simulink model "fin_simu_continuous"  (R2022a)
settings: Solver=ode45  StartTime=0.0  StopTime=time  RelTol=1e-8  AbsTol=1e-10
values from neighbouring files (symbols this model uses):
  A0 = [0, 1; -1, -1.4]    [code_simu_continuous_simplified.m]    (also in matlab.mat = [0  1; -1  -1.4])
  AA_s = [-2.2  -10.2  -9; 1  0  0; 0  1  0]    [matlab.mat]
  AT = [0,1;-9,-1.2]    [code_simu.m]    (also in code_simu_continuous_simplified.m = [0, 1; -9, -1.2]; matlab.mat = [0  1; -9  -1.2])
  b0 = readmatrix('result_NNFF&ROB\20251002_153045\z2_biases_layer_0.csv','Range','A1:A30')    [getNN_simu.m]    (also in matlab.mat = [0.168317809701 -0.0711987838149 -0.0412988699973 -0.0729310)
  B0 = [0; 1]    [code_simu_continuous_simplified.m]    (also in matlab.mat = [0 1])
  b1 = readmatrix('result_NNFF&ROB\20251002_153045\z2_biases_layer_1.csv','Range','A1:A20')    [getNN_simu.m]    (also in matlab.mat = [-0.0446465238929 0.0289220847189 -0.0468313358724 -0.028365)
  b2 = readmatrix('result_NNFF&ROB\20251002_153045\z2_biases_layer_2.csv','Range','A1:A10')    [getNN_simu.m]    (also in matlab.mat = [-0.0184617917985 -0.0854043364525 -0.0408402681351 0.561344)
  b3 = readmatrix('result_NNFF&ROB\20251002_153045\z2_biases_layer_3.csv','Range','A1:A1')    [getNN_simu.m]    (also in matlab.mat = 0.3782748878)
  BB_s = [1 0 0]    [matlab.mat]
  BT = [0;1]    [code_simu.m]    (also in code_simu_continuous_simplified.m = [0; 1]; matlab.mat = [0 1])
  C0 = [1, 0]    [code_simu_continuous_simplified.m]    (also in matlab.mat = [1 0])
  CC_s = [-8.1 -30.42 -14.4]    [matlab.mat]
  CT = [22.5,9]    [code_simu.m]    (also in code_simu_continuous_simplified.m = [22.5, 9]; matlab.mat = [22.5 9])
  D0 = [0]    [code_simu_continuous_simplified.m]    (also in matlab.mat = 0)
  DD_s = 0.1    [matlab.mat]
  DT = 0    [code_simu.m]    (also in code_simu_continuous_simplified.m; matlab.mat)
  gamma = 2    [code_simu.m]    (also in code_simu_continuous_simplified.m = 1000; matlab.mat = 1000)
  omega = 3.14159265*5    (= 15.70796325)    [code_simu.m]    (also in code_simu_continuous_simplified.m; matlab.mat)
  ran_max = 20    [code_simu.m]    (also in code_simu_continuous_simplified.m; matlab.mat)
  ran_min = 5    [code_simu.m]    (also in code_simu_continuous_simplified.m; matlab.mat)
  rho = 0.101    [code_simu.m]    (also in code_simu_continuous_simplified.m = 0.3; matlab.mat = 0.5)
  seed = 17    [code_simu.m]    (also in code_simu_continuous_simplified.m = randi(2^31-2); matlab.mat = 2084332126)
  sigma = 10    [code_simu.m]    (also in code_simu_continuous_simplified.m = 0.1; matlab.mat = 100)
  Td = 0.001    [code_simu_continuous_simplified.m]    (also in matlab.mat)
  w0 = readmatrix('result_NNFF&ROB\20251002_153045\z2_weights_layer_0.csv','Range','A1:AD4')    [getNN_simu.m]    (also in matlab.mat = [0.408856898546 -0.0425847135484 0.404223948717 0.4036423563)
  w1 = readmatrix('result_NNFF&ROB\20251002_153045\z2_weights_layer_1.csv','Range','A1:T30')    [getNN_simu.m]    (also in matlab.mat = [0.0375822260976 -0.0405062437057 0.109349139035 0.202072694)
  w2 = readmatrix('result_NNFF&ROB\20251002_153045\z2_weights_layer_2.csv','Range','A1:J20')    [getNN_simu.m]    (also in matlab.mat = [-0.29533213377 -0.372659087181 -0.239123016596 0.2688936889)
  w3 = readmatrix('result_NNFF&ROB\20251002_153045\z2_weights_layer_3.csv','Range','A1:A10')    [getNN_simu.m]    (also in matlab.mat = [0.481317937374 0.267534017563 -0.184389919043 -0.8444167971)
  wav = 0.7    [code_simu.m]    (also in code_simu_continuous_simplified.m; matlab.mat)
libraries: simulink x1
settings Model: Creator=IDS_PC  LastModifiedBy=IDS_PC
settings SolverCC: SolverResetMethod=Robust
settings DebuggingCC: AlgebraicLoopMsg=none

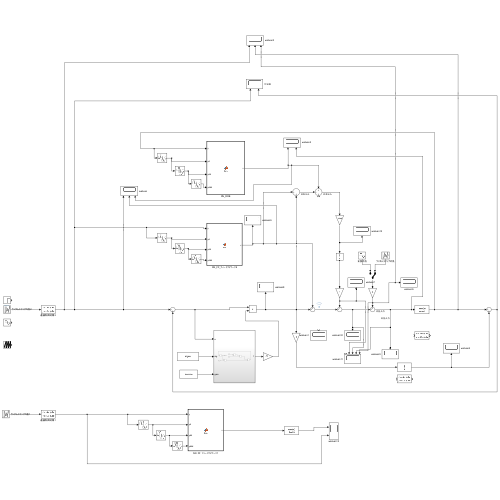
[thumbnail: Simulink's stored preview of the top-level diagram]
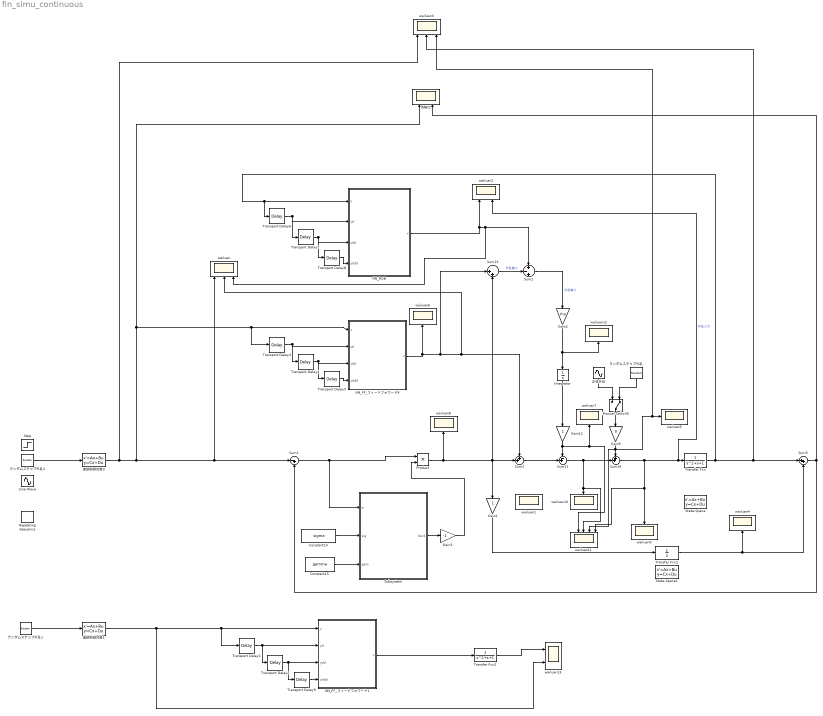
== system fin_simu_continuous ==
  " 正弦外乱" : Sin  Amplitude=wav  Bias=1  Frequency=omega  Phase=1  SampleTime=0
  Constant14 : Constant  Value=sigma  SampleTime=0
  Constant15 : Constant  Value=gamma  SampleTime=0
  Gain1 : Gain
  Gain12 : Gain
  Gain2 : Gain  Gain=rho
  Gain3 : Gain  Gain=-1
  Gain5 : Gain  Gain=0
  Integrator : Integrator
  Manual Switch5 : ManualSwitch  CurrentSetting=0
  NN_FF_フィードフォワード1 : MATLAB Function  TreatAsAtomicUnit=on
  NN_FF_フィードフォワード9 : MATLAB Function  TreatAsAtomicUnit=on
  NN_ROB : MATLAB Function  TreatAsAtomicUnit=on
  Product : Product
  Repeating Sequence : simulink/Sources/Repeating Sequence  rep_seq_t=[0 2]  rep_seq_y=[0 2]
  Sine Wave : Sin  SampleTime=0
  State-Space : StateSpace  A=AT  B=BT  C=CT  D=DT  InitialCondition=0
  State-Space1 : StateSpace  A=AA_s  B=BB_s  C=CC_s  D=DD_s  InitialCondition=0
  Step : Step  SampleTime=0
  Subsystem : Subsystem
  Sum1 : Sum  Inputs=|-+
  Sum11 : Sum  Inputs=-+|
  Sum13 : Sum  Inputs=|++
  Sum16 : Sum  Inputs=++|
  Sum2 : Sum  Inputs=+-+
  Sum3 : Sum  Inputs=++|
  Sum5 : Sum  Inputs=|++
  Transfer Fcn : TransferFcn  Denominator=[1 1 1]
  Transfer Fcn1 : TransferFcn  Denominator=[2]
  Transfer Fcn2 : TransferFcn  Denominator=[1 1 1]
  Transport Delay{1..9} (9 alike) : TransportDelay  DelayTime=Td
  wailuan : Scope  NumInputPorts=3
  wailuan{1,4..10,12} (9 alike) : Scope
  wailuan11 : Scope  NumInputPorts=5
  wailuan13 : Scope  NumInputPorts=2
  wailuan2 : Scope  NumInputPorts=2
  wailuan3 : Scope  NumInputPorts=3
  ランダムステップ外乱 : UniformRandomNumber  Minimum=-wav  Maximum=wav  Seed=seed  SampleTime=16
  ランダムステップ外乱1 : UniformRandomNumber  Minimum=ran_min  Maximum=ran_max  Seed=seed  SampleTime=32
  ランダムステップ外乱2 : UniformRandomNumber  Minimum=ran_min  Maximum=ran_max  Seed=seed  SampleTime=32
  伪输出 : Scope  NumInputPorts=2
  連続制御対象1 : StateSpace  A=A0  B=B0  C=C0  D=D0  InitialCondition=0
  連続制御対象3 : StateSpace  A=A0  B=B0  C=C0  D=D0  InitialCondition=0
  wires:
  Sum16/1 -> wailuan2/2, Transfer Fcn/1, wailuan11/5, wailuan9/1  "外乱入力"
  Gain5/1 -> wailuan11/4, wailuan3/3, wailuan5/1, Sum16/1
  Manual Switch5/1 -> Gain5/1
  ランダムステップ外乱/1 -> Manual Switch5/2
  " 正弦外乱"/1 -> Manual Switch5/1
  Sum11/1 -> Sum16/2, wailuan11/3, wailuan10/1
  Gain12/1 -> Sum11/1, wailuan11/2, wailuan7/1
  Product/1 -> Gain1/1, Sum3/2, Sum13/2, wailuan8/1
  Transfer Fcn/1 -> wailuan3/2, Sum5/1, Transport Delay6/1, NN_ROB/1(y)
  連続制御対象3/1 -> wailuan3/1, Sum1/1, wailuan/1, 伪输出/1, Transport Delay3/1, NN_FF_フィードフォワード9/1(y)
  NN_FF_フィードフォワード9/1(v) -> wailuan/2, Sum3/1, Sum13/1, wailuan6/1
  NN_ROB/1(v) -> wailuan/3, Sum2/1, wailuan2/1
  Sum13/1 -> Sum2/2  "外乱输入"
  Gain2/1 -> wailuan12/1, Integrator/1
  Sum2/1 -> Gain2/1  "外乱输入"
  Integrator/1 -> Gain12/1
  Transport Delay5/1 -> NN_FF_フィードフォワード9/4(yddd)
  Transport Delay4/1 -> Transport Delay5/1, NN_FF_フィードフォワード9/3(ydd)
  Transport Delay3/1 -> Transport Delay4/1, NN_FF_フィードフォワード9/2(yd)
  Transport Delay8/1 -> NN_ROB/4(yddd)
  Transport Delay6/1 -> Transport Delay7/1, NN_ROB/2(yd)
  Transport Delay7/1 -> Transport Delay8/1, NN_ROB/3(ydd)
  Gain1/1 -> Transfer Fcn1/1
  Transfer Fcn1/1 -> Sum5/2, wailuan4/1
  ランダムステップ外乱2/1 -> 連続制御対象3/1
  Sum5/1 -> 伪输出/2, Sum1/2
  Sum1/1 -> Product/1, Subsystem/1(e)
  Constant14/1 -> Subsystem/2(sig)
  Constant15/1 -> Subsystem/3(gam)
  Subsystem/1(Out1) -> Gain3/1
  Gain3/1 -> Product/2
  Sum3/1 -> Sum11/2
  ランダムステップ外乱1/1 -> 連続制御対象1/1
  連続制御対象1/1 -> wailuan13/2, Transport Delay1/1, NN_FF_フィードフォワード1/1(y)
  Transport Delay9/1 -> NN_FF_フィードフォワード1/4(yddd)
  Transport Delay2/1 -> Transport Delay9/1, NN_FF_フィードフォワード1/3(ydd)
  Transport Delay1/1 -> Transport Delay2/1, NN_FF_フィードフォワード1/2(yd)
  NN_FF_フィードフォワード1/1(v) -> Transfer Fcn2/1
  Transfer Fcn2/1 -> wailuan13/1

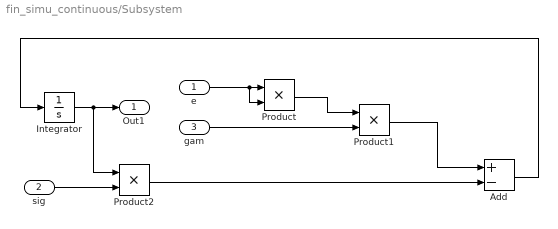
== system fin_simu_continuous/Subsystem ==
  e : Inport
  sig : Inport  Port=2
  gam : Inport  Port=3
  Add : Sum  Inputs=+-
  Integrator : Integrator  UpperSaturationLimit=999999999999999999  LowerSaturationLimit=-9999999999999999
  Product : Product
  Product1 : Product
  Product2 : Product
  Out1 : Outport
  wires:
  e/1 -> Product/2, Product/1
  Product/1 -> Product1/1
  gam/1 -> Product1/2
  Integrator/1 -> Product2/1, Out1/1
  sig/1 -> Product2/2
  Product2/1 -> Add/2
  Product1/1 -> Add/1
  Add/1 -> Integrator/1

== matlab function fin_simu_continuous/NN_ROB ==
  data: y input; yd input; ydd input; yddd input; v output; w0 parameter; w1 parameter; w2 parameter; w3 parameter; b0 parameter; b1 parameter; b2 parameter; b3 parameter
function v = fcn(y, yd, ydd, yddd, w0, w1, w2, w3, b0, b1, b2, b3)

    x = [y, yd, ydd, yddd];
    x = x.';

    s1= (transpose(w0)) * x + b0;
    x1= max(0,s1);     %relu 
    s2= (transpose(w1)) * x1 + b1;
    x2= max(0,s2);     %relu
    s3= (transpose(w2)) * x2 + b2;
    x3= max(0,s3);     %relu
    s4= (transpose(w3)) * x3 + b3;

v=s4;

== matlab function fin_simu_continuous/NN_FF_フィードフォワード1 ==
  data: y input; yd input; ydd input; yddd input; v output; w0 parameter; w1 parameter; w2 parameter; w3 parameter; b0 parameter; b1 parameter; b2 parameter; b3 parameter
function v = fcn(y, yd, ydd, yddd, w0, w1, w2, w3, b0, b1, b2, b3)

    x = [yddd, ydd, yd, y];
    x = x.';

    s1= (transpose(w0)) * x + b0;
    x1= max(0,s1);     %relu 
    s2= (transpose(w1)) * x1 + b1;
    x2= max(0,s2);     %relu
    s3= (transpose(w2)) * x2 + b2;
    x3= max(0,s3);     %relu
    s4= (transpose(w3)) * x3 + b3;

v=s4;

== matlab function fin_simu_continuous/NN_FF_フィードフォワード9 ==
  data: y input; yd input; ydd input; yddd input; v output; w0 parameter; w1 parameter; w2 parameter; w3 parameter; b0 parameter; b1 parameter; b2 parameter; b3 parameter
function v = fcn(y, yd, ydd, yddd, w0, w1, w2, w3, b0, b1, b2, b3)

    x = [y, yd, ydd, yddd];
    x = x.';

    s1= (transpose(w0)) * x + b0;
    x1= max(0,s1);     %relu 
    s2= (transpose(w1)) * x1 + b1;
    x2= max(0,s2);     %relu
    s3= (transpose(w2)) * x2 + b2;
    x3= max(0,s3);     %relu
    s4= (transpose(w3)) * x3 + b3;

v=s4;
